simulink model "inverted_pendulum"  (R2023a)
settings: Solver=VariableStepAuto  StartTime=0.0  StopTime=50  RelTol=1e-3
values from neighbouring files (symbols this model uses):
  d_theta_init = 0    [parameters_inv_pend.m]
  d_x_init = 0    [parameters_inv_pend.m]
  g = 9.81    [parameters_inv_pend.m]
  l = 1    [parameters_inv_pend.m]
  M = 1    [parameters_inv_pend.m]
  m = .1    (= 0.1)    [parameters_inv_pend.m]
  theta_init = .3    (= 0.3)    [parameters_inv_pend.m]
  x_init = 0    [parameters_inv_pend.m]
libraries: fuzblock x1
settings Model: Creator=luand  LastModifiedBy=luand

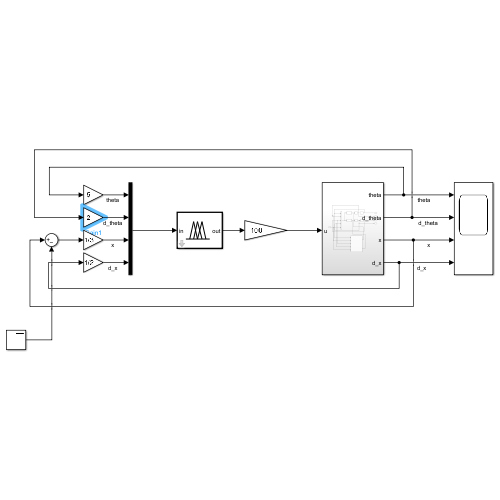
[thumbnail: Simulink's stored preview of the top-level diagram]
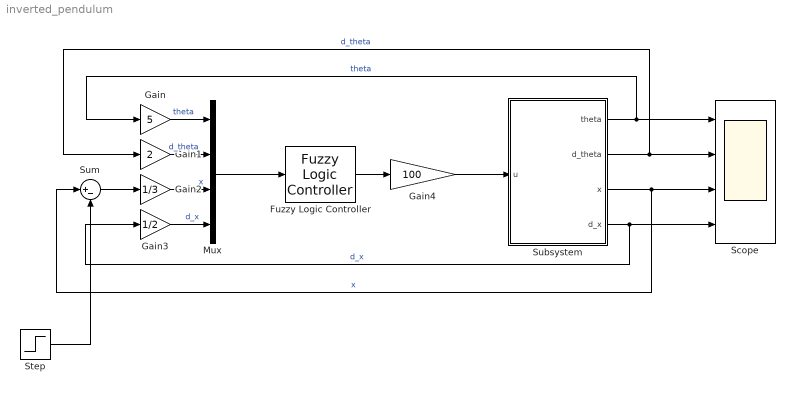
== system inverted_pendulum ==
  Fuzzy Logic Controller : fuzblock/Fuzzy Logic  Controller  FIS='fuzzy_angle.fis'  OutputSampleNumber=101  DataType=double  FuzzifiedInputs=off  RuleFiringStrengths=off  RuleOutputs=off  AggregatedOutputs=off  SimulateUsing=Interpreted execution  OutOfRangeInputValueMessage=warning  NoRuleFiredMessage=warning  EmptyOutputFuzzySetMessage=warning
  Gain : Gain  Gain=5
  Gain1 : Gain  Gain=2
  Gain2 : Gain  Gain=1/3
  Gain3 : Gain  Gain=1/2
  Gain4 : Gain  Gain=100
  Mux : Mux
  Scope : Scope  NumInputPorts=4
  Step : Step  Time=50  After=.3  SampleTime=0
  Subsystem : Subsystem
  Sum : Sum  Inputs=|+-
  wires:
  Subsystem/1(theta) -> Gain/1, Scope/1  "theta"
  Subsystem/2(d_theta) -> Gain1/1, Scope/2  "d_theta"
  Subsystem/3(x) -> Sum/1, Scope/3  "x"
  Subsystem/4(d_x) -> Gain3/1, Scope/4  "d_x"
  Mux/1 -> Fuzzy Logic Controller/1
  Fuzzy Logic Controller/1 -> Gain4/1
  Gain/1 -> Mux/1  "theta"
  Gain1/1 -> Mux/2  "d_theta"
  Gain2/1 -> Mux/3  "x"
  Gain3/1 -> Mux/4  "d_x"
  Gain4/1 -> Subsystem/1(u)
  Step/1 -> Sum/2
  Sum/1 -> Gain2/1

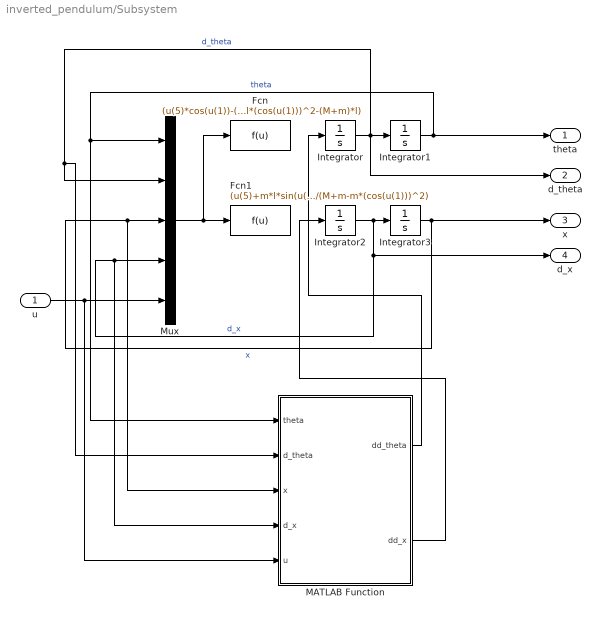
== system inverted_pendulum/Subsystem ==
  u : Inport
  Fcn : Fcn  Expr=(u(5)*cos(u(1))-(M+m)*g*sin(u(1))+m*l*cos(u(1))*sin(u(1))*u(2))/(m*l*(cos(u(1)))^2-(M+m)*l)
  Fcn1 : Fcn  Expr=(u(5)+m*l*sin(u(2))*(u(2))^2-m*g*cos(u(1))*sin(u(1)))/(M+m-m*(cos(u(1)))^2)
  Integrator : Integrator  InitialCondition=d_theta_init
  Integrator1 : Integrator  InitialCondition=theta_init
  Integrator2 : Integrator  InitialCondition=d_x_init
  Integrator3 : Integrator  InitialCondition=x_init
  MATLAB Function : MATLAB Function  TreatAsAtomicUnit=on
  Mux : Mux  Inputs=5
  theta : Outport
  d_theta : Outport  Port=2
  x : Outport  Port=3
  d_x : Outport  Port=4
  wires:
  u/1 -> MATLAB Function/5(u), Mux/5
  Mux/1 -> Fcn1/1, Fcn/1
  Integrator/1 -> d_theta/1, MATLAB Function/2(d_theta), Mux/2, Integrator1/1  "d_theta"
  Integrator1/1 -> MATLAB Function/1(theta), Mux/1, theta/1  "theta"
  Integrator2/1 -> MATLAB Function/4(d_x), Mux/4, d_x/1, Integrator3/1  "d_x"
  Integrator3/1 -> MATLAB Function/3(x), Mux/3, x/1  "x"
  MATLAB Function/1(dd_theta) -> Integrator/1
  MATLAB Function/2(dd_x) -> Integrator2/1

== matlab function inverted_pendulum/Subsystem/MATLAB Function ==
  data: dd_theta output; theta input; d_theta input; x input; d_x input; u input; dd_x output
function [dd_theta,dd_x] = fcn(theta, d_theta, x, d_x, u)
M = 1; m = .1; l = 1; g = 9.81;

theta_init = .01;
d_theta_init = 0;

x_init = .02;
d_x_init = 0;

dd_theta =(u*cos(theta)-(M+m)*g*sin(theta)+m*l*cos(theta)*sin(theta)*d_theta)/(m*l*(cos(theta))^2-(M+m)*l)
dd_x = (u+m*l*sin(theta)*(d_theta)^2-m*g*cos(theta)*sin(theta))/(M+m-m*(cos(theta))^2)
%dd_x = (m*g*sin(theta)-m*l*dd_theta)/(m*cos(theta))
